simulink subsystem "GMST_angle_from_datetime"  (R2022a)
settings: Solver=VariableStepAuto  StartTime=0.0  StopTime=10.0  RelTol=1e-3
settings Model: Creator=samuel  LastModifiedBy=samuel

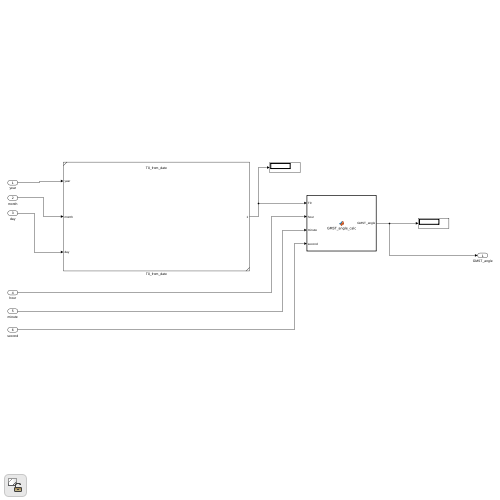
[thumbnail: Simulink's stored preview of the top-level diagram]
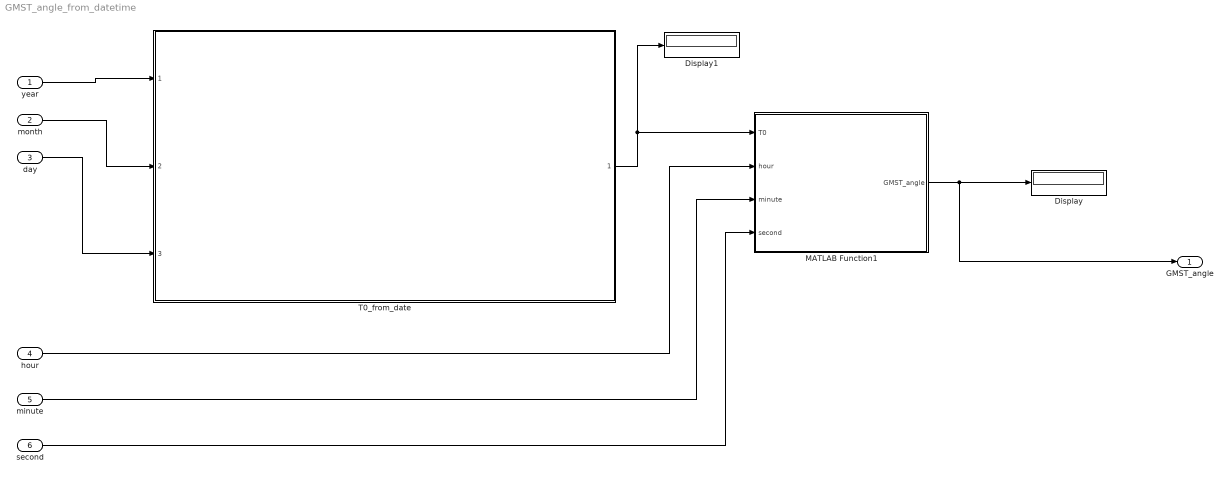
== system GMST_angle_from_datetime ==
  year : Inport
  month : Inport  Port=2
  day : Inport  Port=3
  hour : Inport  Port=4
  minute : Inport  Port=5
  second : Inport  Port=6
  Display : Display
  Display1 : Display
  MATLAB Function1 : MATLAB Function  TreatAsAtomicUnit=on
  T0_from_date : Subsystem  ReferencedSubsystem=T0_from_date
  GMST_angle : Outport
  wires:
  second/1 -> MATLAB Function1/4(second)
  hour/1 -> MATLAB Function1/2(hour)
  T0_from_date/1 -> MATLAB Function1/1(T0), Display1/1
  MATLAB Function1/1(GMST_angle) -> Display/1, GMST_angle/1
  month/1 -> T0_from_date/2
  year/1 -> T0_from_date/1
  minute/1 -> MATLAB Function1/3(minute)
  day/1 -> T0_from_date/3

== matlab function GMST_angle_from_datetime/MATLAB Function1 ==
  data: T0 input; GMST_angle output; hour input; minute input; second input
function GMST_angle = GMST_angle_calc(T0, hour, minute, second)
    GMST_angle_temp = 24110.54841 + 8640184.812866 * ...
        T0 + 0.0931104 * T0^2 - 6.2e-6*T0^3 + ...
        1.002737909350795*(3600*hour + 60*minute + second);

    % we need to add/subtract 68400 to get to the range of 0 to 86400
    % seconds (longitudinal seconds), this is accomplished easily with mod

    GMST_angle_temp = mod(GMST_angle_temp, 86400);
    
    % longitudinal seconds are 1/240 degrees, want to convert back
    GMST_angle = GMST_angle_temp / 240;
